simulink model "HornetXII_Challenge"  (R2026a)
settings: Solver=VariableStepAuto  StopTime=300  AbsTol=1e-3  EnableMultiTasking=on
InitFcn:
  | searchHalfSpan = 5;
  | 
  | rng('shuffle');
  | Environment.target.seed = randi(2^31 - 1);
  | 
  | % Use the saved seed to make this particular run reproducible if needed.
  | rng(Environment.target.seed, 'twister');
  | 
  | Environment.target.xy = (2*rand(2,1) - 1) * searchHalfSpan;
  | 
  | Environment.target.pos = [Environment.target.xy;
  |     Environment.seafloordepth - Environment.target.side/2];
values from neighbouring files (symbols this model uses):
  N = size(Vehicle.thrusterori, 2)    [VehicleParameters.m]
undefined symbols (not defined in the file or in its folder): B, pospoints, Spline, timepoints, Vehicle, X, Y, Z
libraries: sm_lib x554, nesl_utility x23, slpidlib x13, matrix_library x4, robotcorelib x2, fl_lib x1, simulink x1
(part 1 of 14)
settings Model: Creator=chesi  LastModifiedBy=kianm
settings DebuggingCC: SubsystemReferenceDiagnosticForUnitTest=warning
settings SimscapeCC: SimscapeNominalValues="[{\"value\":\"1\",\"unit\":\"A\"},{\"value\":\"1\",\"unit\":\"bar\"},{\"value\":\"1\",\"unit\":\"cm^2\"},{\"value\":\"1\",\"unit\":\"cm^3/s\"},{\"value\":\"1\",\"unit\":\"kJ/kg\"},{\"value\":\"1\",\"unit\":\"kW\"},{\"value\":\"1\",\"unit\":\"l\"},{\"value\":\"1\",\"unit\":\"N\"},{\"value\":\"1\",\"unit\":\"N*m\"},{\"value\":\"1\",\"unit\":\"V\"}]"  SimscapeLogSimulationStatistics=on
settings ExplorerConfigSet: InternalSimMechanicsExplorerSettings=|
  | <ExplorerConfiguration>
  | 
  |   <canonicalview>default</canonicalview>
  | 
  |   <TilePanel>
  |     <TileInfo>
  |       <Tiles Columns="2" Count="4" Height="1049" Rows="2" Width="1462">
  |         <Row Weight="0.5"/>
  |         <Row Weight="0.5"/>
  |         <Column Weight="0.5"/>
  |         <Column Weight="0.5"/>
  |         <Tile Height="1" Width="1" X="0" Y="0"/>
  |         <Tile Height="1" Width="1" X="0" Y="1"/>
  |         <Tile Height="1" Width="1" X="1" Y="0"/>
  |         <Tile Height="1" Width="1" X="1" Y="1"/>
  |       </Tiles>
  |     </TileInfo>
  |     <SceneInfo>
  |       <SceneViewer>
  |         <IsThisViewStd>
  |           <IsStandardView>off</IsStandardView>
  |           <StandardViewName>Front</StandardViewName>
  |         </IsThisViewStd>
  |         <BGColor>
  |           <R>1</R>
  |           <G>1</G>
  |           <B>1</B>
  |           <A>1</A>
  |         </BGColor>
  |         <Camera>
  |           <DoPerspective>on</DoPerspective>
  |           <Position>
  |             <X>-1.4139999999999999</X>
  |             <Y>0</Y>
  |             <Z>1</Z>
  |           </Position>
  |           <Center>
  |             <X>0</X>
  |             <Y>0</Y>
  |             <Z>0</Z>
  |           </Center>
  |           <Up>
  |             <X>0.57740839789430587</X>
  |             <Y>0</Y>
  |             <Z>0.81645547462254864</Z>
  |           </Up>
  |           <XLim>0.80758724648884639</XLim>
  |           <YLim>0.80758724648884639</YLim>
  |           <ViewLimDist>0.01</ViewLimDist>
  |         </Camera>
  |       </SceneViewer>
  |       <SceneViewer>
  |         <IsThisViewStd>
  |           <IsStandardView>off</IsStandardView>
  |           <StandardViewName>Front</StandardViewName>
  |         </IsThisViewStd>
  |         <BGColor>
  |           <R>1</R>
  |           <G>1</G>
  |           <B>1</B>
  |           <A>1</A>
  |         </BGColor>
  |         <Camera>
  |           <DoPerspective>on</DoPerspective>
  |           <Position>
  |             <X>0</X>
  |             <Y>0</Y>
  |             <Z>2.5</Z>
  |           </Position>
  |           <Center>
  |             <X>0</X>
  |             <Y>0</Y>
  |             <Z>0</Z>
  |           </Center>
  |           <Up>
  |             <X>1</X>
  |             <Y>0</Y>
  |             <Z>0</Z>
  |           </Up>
  |           <XLim>1.1657691453874972</XLim>
  |           <YLim>1.1657691453874972</YLim>
  |           <ViewLimDist>0.01</ViewLimDist>
  |         </Camera>
  |       </SceneViewer>
  |       <SceneViewer>
  |         <IsThisViewStd>
  |           <IsStandardView>off</IsStandardView>
  |           <StandardViewName>Front</StandardViewName>
  |         </IsThisViewStd>
  |         <BGColor>
  |           <R>1</R>
  |           <G>1</G>
  |           <B>1</B>
  |           <A>1</A>
  |         </BGColor>
  |         <Camera>
  |           <DoPerspective>off</DoPerspective>
  |           <Position>
  |             <X>-0.023481336045726414</X>
  |             <Y>1.0064517868689387</Y>
  |             <Z>83.52507923435725</Z>
  |           </Position>
  |           <Center>
  |             <X>-0.010188562910498078</X>
  |             <Y>1</Y>
  |             <Z>-1.4383130630604528</Z>
  |           </Center>
  |           <Up>
  |             <X>0.99999998774834031</X>
  |             <Y>5.0907915827116125e-06</Y>
  |             <Z>0.00015645255878126614</Z>
  |           </Up>
  |           <XLim>10.310637364602009</XLim>
  |           <YLim>10.310637364602009</YLim>
  |           <ViewLimDist>0.01</ViewLimDist>
  |         </Camera>
  |       </SceneViewer>
  |       <SceneViewer>
  |         <IsThisViewStd>
  |           <IsStandardView>off</IsStandardView>
  |           <StandardViewName>Front</StandardViewName>
  |         </IsThisViewStd>
  |         <BGColor>
  |           <R>1</R>
  |           <G>1</G>
  |           <B>1</B>
  |           <A>1</A>
  |         </BGColor>
  |         <Camera>
  |           <DoPerspective>on</DoPerspective>
  |           <Position>
  |             <X>0</X>
  |             <Y>0</Y>
  |             <Z>-0.25</Z>
  |           </Position>
  |           <Center>
  |             <X>0</X>
  |             <Y>0</Y>
  |             <Z>-1.25</Z>
  |           </Center>
  |           <Up>
  |             <X>1</X>
  |             <Y>0</Y>
  |             <Z>0</Z>
  |           </Up>
  |           <XLim>0.46630765815499897</XLim>
  |           <YLim>0.46630765815499897</YLim>
  |           <ViewLimDist>0.01</ViewLimDist>
  |         </Camera>
  |       </SceneViewer>
  |     </SceneInfo>
  |   </TilePanel>
  | 
  |   <MechEditorPanel>
  |     <GfxPanelCameraMap>
  |       <MapElement CameraMLId="Camera5" GfxPanelIndex="0"/>
  |       <MapElement CameraMLId="Camera7" GfxPanelIndex="1"/>
  |       <MapElement CameraMLId="Camera9" GfxPanelIndex="3"/>
  |     </GfxPanelCameraMap>
  |     <Cameras>
  |       <Camera>
  |         <Id>Camera5</Id>
  |         <Value>
  |           <Name>Behind Up</Name>
  |           <NativeCamera>
  |             <PositionTrackingFeature>Simulator.Cameras.Behind_Up.R</PositionTrackingFeature>
  |             <CenterTrackingFeature>Simulator.AUV_model.BODY</CenterTrackingFeature>
  |             <UpVectorTrackingFeature>Simulator.AUV_model.BODY</UpVectorTrackingFeature>
  |             <CenterTrackingOrigin>on</CenterTrackingOrigin>
  |             <UpVectorTrackingDirection>+X</UpVectorTrackingDirection>
  |           </NativeCamera>
  |         </Value>
  |       </Camera>
  |       <Camera>
  |         <Id>Camera6</Id>
  |         <Value>
  |           <Name>Behind Up Left</Name>
  |           <NativeCamera>
  |             <PositionTrackingFeature>Simulator.Cameras.Behind_Up_Left.R</PositionTrackingFeature>
  |             <CenterTrackingFeature>Simulator.AUV_model.BODY</CenterTrackingFeature>
  |             <UpVectorTrackingFeature>Simulator.AUV_model.BODY</UpVectorTrackingFeature>
  |             <CenterTrackingOrigin>on</CenterTrackingOrigin>
  |             <UpVectorTrackingDirection>-Z</UpVectorTrackingDirection>
  |           </NativeCamera>
  |         </Value>
  |       </Camera>
  |       <Camera>
  |         <Id>Camera7</Id>
  |         <Value>
  |           <Name>Top</Name>
  |           <NativeCamera>
  |             <PositionTrackingFeature>Simulator.Cameras.Top.R</PositionTrackingFeature>
  |             <CenterTrackingFeature>Simulator.AUV_model.BODY</CenterTrackingFeature>
  |             <UpVectorTrackingFeature>Simulator.AUV_model.BODY</UpVectorTrackingFeature>
  |             <CenterTrackingOrigin>on</CenterTrackingOrigin>
  |             <UpVectorTrackingDirection>+X</UpVectorTrackingDirection>
  |           </NativeCamera>
  |         </Value>
  |       </Camera>
  |       <Camera>
  |         <Id>Camera8</Id>
  |         <Value>
  |           <Name>Left</Name>
  |           <NativeCamera>
  |             <PositionTrackingFeature>Simulator.Cameras.Left.R</PositionTrackingFeature>
  |             <CenterTrackingFeature>Simulator.AUV_model.BODY</CenterTrackingFeature>
  |             <UpVectorTrackingFeature>Simulator.AUV_model.BODY</UpVectorTrackingFeature>
  |             <CenterTrackingOrigin>on</CenterTrackingOrigin>
  |             <UpVectorTrackingDirection>-Z</UpVectorTrackingDirection>
  |           </NativeCamera>
  |         </Value>
  |       </Camera>
  |       <Camera>
  |         <Id>Camera9</Id>
  |         <Value>
  |           <Name>BottomCamera</Name>
  |           <NativeCamera>
  |             <PositionTrackingFeature>Simulator.Cameras.Bottom_Camera.R</PositionTrackingFeature>
  |             <CenterTrackingFeature>Simulator.Cameras.Bottom_Camera.R</CenterTrackingFeature>
  |             <UpVectorTrackingFeature>Simulator.Cameras.Bottom_Camera.R</UpVectorTrackingFeature>
  |             <CenterTrackingOrigin>off</CenterTrackingOrigin>
  |             <CenterTrackingDirection>+Z</CenterTrackingDirection>
  |             <UpVectorTrackingDirection>+X</UpVectorTrackingDirection>
  |           </NativeCamera>
  |         </Value>
  |       </Camera>
  |     </Cameras>
  |     <VideoCreator>
  |       <IncludeTiles>All</IncludeTiles>
  |       <IncludeTime>on</IncludeTime>
  |       <IncludeWorldFrame>off</IncludeWorldFrame>
  |       <PlaybackSpeedRatio>1</PlaybackSpeedRatio>
  |       <FrameRate>30</FrameRate>
  |       <FrameSize>auto</FrameSize>
  |       <VideoFormat>UncompressedAVI</VideoFormat>
  |     </VideoCreator>
  |   </MechEditorPanel>
  | 
  |   <PlaybackSettings>
  |     <PlaybackSpeedFactor>2</PlaybackSpeedFactor>
  |   </PlaybackSettings>
  | 
  | </ExplorerConfiguration>

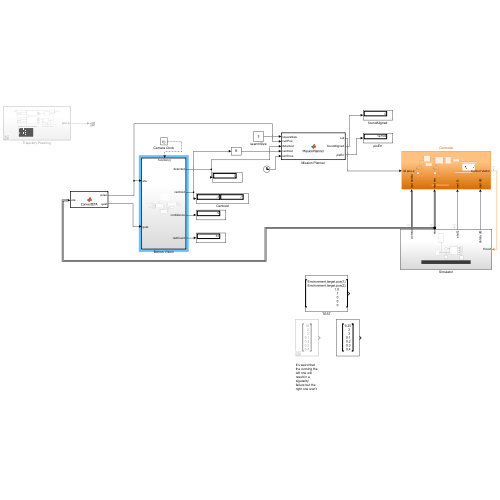
[thumbnail: Simulink's stored preview of the top-level diagram]
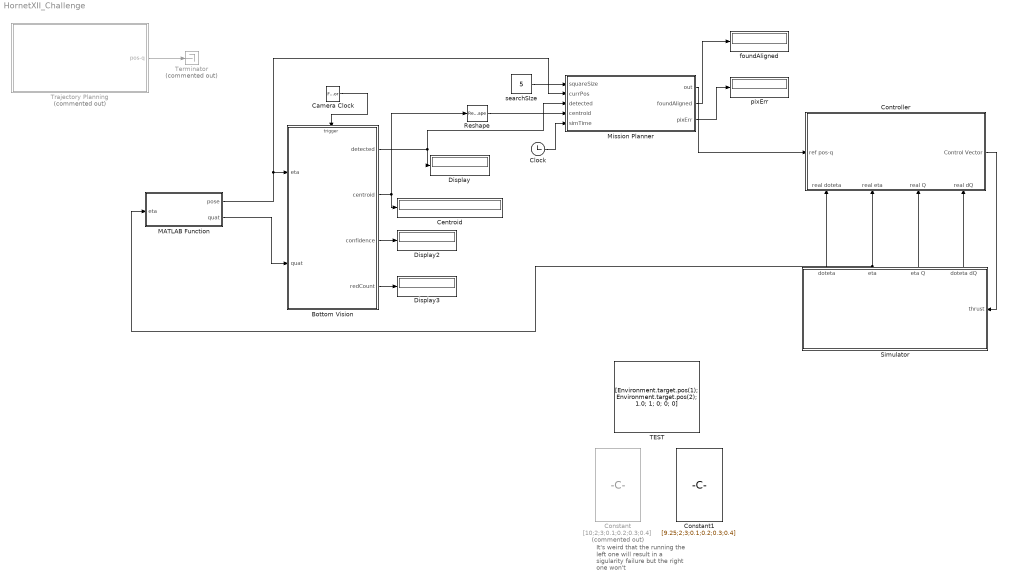
== system HornetXII_Challenge ==
  note: It's weird that the running the left one will result in a sigularity failure but the right one won't
  Bottom Vision : Subsystem  TreatAsAtomicUnit=on
  Camera Clock : FunctionCallGenerator  SampleTime=.2
  Centroid : Display
  Clock : Clock
  Constant : Constant  Commented=on  Value=[10;2;3;0.1;0.2;0.3;0.4]  VectorParams1D=off
  Constant1 : Constant  Value=[9.25;2;3;0.1;0.2;0.3;0.4]  VectorParams1D=off
  Controller : Subsystem
      settings: PortSchema="{\"entries\":[{\"content\":{\"sides\":[{\"content\":{\"connectorIds\":[\"In1\"]},\"type\":\"ConnectorPlacement.EquallySpacedRectSide\",\"uuid\":\"81dc70ea-c00b-487c-98ee-990ff0e578a9\"},{\"content\":{\"connectorIds\":[\"Out1\"],\"side\":\"RIGHT\"},\"type\":\"ConnectorPlacement.EquallySpacedRectSide\",\"uuid\":\"b4d94801-500f-4262-ae87-d28847072c57\"},{\"content\":{\"side\":\"TOP\"},\"type\":\"ConnectorPlacement.EquallySpacedRectSide\",\"uuid\":\"9c8bb19e-0c4f-4865-8be8-8f504c3461c9\"},{\"content\":{\"connectorIds\":[\"In2\",\"In3\",\"In4\",\"In5\"],\"side\":\"BOTTOM\"},\"type\":\"ConnectorPlacement.EquallySpacedRectSide\",\"uuid\":\"42aa0f8d-cdff-4cb2-b13b-82c7b92e497b\"}]},\"type\":\"ConnectorPlacement.EquallySpacedConnector\",\"uuid\":\"3d0765d3-7e16-47e0-887a-613e0e5dbe32\"}],\"packageUris\":[\"http://schema.mathworks.com/mf0/Connector/R2020b\"],\"version\":\"1.0\"}"
  Display : Display
  Display2 : Display
  Display3 : Display
  MATLAB Function : MATLAB Function  TreatAsAtomicUnit=on
  Mission Planner : MATLAB Function  TreatAsAtomicUnit=on
  Reshape : Reshape  OutputDimensionality=Customize  OutputDimensions=[2,1]
  Simulator : Subsystem
      settings: PortSchema="{\"entries\":[{\"content\":{\"sides\":[{\"content\":{\"connectorIds\":[\"In1\"]},\"type\":\"ConnectorPlacement.EquallySpacedRectSide\",\"uuid\":\"7f0b7788-e8a3-4936-9374-02ac1b67f663\"},{\"content\":{\"side\":\"RIGHT\"},\"type\":\"ConnectorPlacement.EquallySpacedRectSide\",\"uuid\":\"45623c25-ae9c-4192-a7b0-dfa9bedf06ea\"},{\"content\":{\"connectorIds\":[\"Out1\",\"Out2\",\"Out3\",\"Out4\"],\"side\":\"TOP\"},\"type\":\"ConnectorPlacement.EquallySpacedRectSide\",\"uuid\":\"6471b253-20e0-4344-8e89-5b5e84cfa395\"},{\"content\":{\"side\":\"BOTTOM\"},\"type\":\"ConnectorPlacement.EquallySpacedRectSide\",\"uuid\":\"e37f05fa-5476-47a4-acd2-111dd632b18c\"}]},\"type\":\"ConnectorPlacement.EquallySpacedConnector\",\"uuid\":\"72a4f9be-cf7b-4481-94c8-675ac13ca12c\"}],\"packageUris\":[\"http://schema.mathworks.com/mf0/Connector/R2020b\"],\"version\":\"1.0\"}"
  TEST : Constant  Value=|  VectorParams1D=off
      | [Environment.target.pos(1);
      |  Environment.target.pos(2);
      |  1.0;
      |  1;
      |  0;
      |  0;
      |  0]
  Terminator : Terminator  Commented=on
  Trajectory Planning : Subsystem  Commented=on
  foundAligned : Display
  pixErr : Display
  searchSIze : Constant  Value=5
  wires:
  searchSIze/1 -> Mission Planner/1(squareSize)
  Trajectory Planning/1(pos-q) -> Terminator/1
  Simulator/4(doteta) -> Controller/2(real doteta)
  Simulator/2(eta Q) -> Controller/4(real Q)
  MATLAB Function/2(quat) -> Bottom Vision/2(quat)
  Simulator/3(eta) -> Controller/3(real eta), MATLAB Function/1(eta)
  Simulator/1(doteta dQ) -> Controller/5(real dQ)
  Camera Clock/1 -> Bottom Vision/Trigger
  MATLAB Function/1(pose) -> Mission Planner/2(currPos), Bottom Vision/1(eta)
  Bottom Vision/3(confidence) -> Display2/1
  Bottom Vision/1(detected) -> Mission Planner/3(detected), Display/1
  Bottom Vision/4(redCount) -> Display3/1
  Bottom Vision/2(centroid) -> Reshape/1, Centroid/1
  Reshape/1 -> Mission Planner/4(centroid)
  Clock/1 -> Mission Planner/5(simTime)
  Mission Planner/1(out) -> Controller/1(ref pos-q)
  Mission Planner/2(foundAligned) -> foundAligned/1
  Mission Planner/3(pixErr) -> pixErr/1
  Controller/1(Control Vector) -> Simulator/1(thrust)

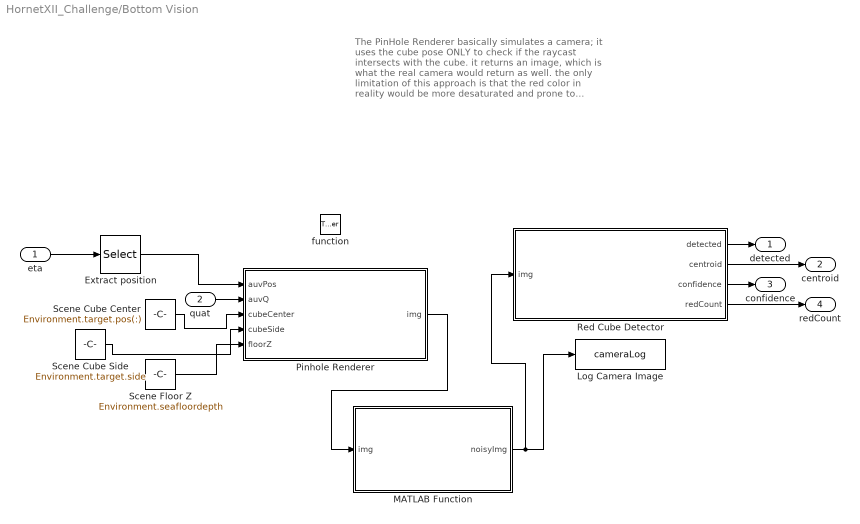
== system HornetXII_Challenge/Bottom Vision ==
  note: The PinHole Renderer basically simulates a camera; it uses the cube pose ONLY to check if the raycast intersects with the cube. it returns an image, which is what the real camera would return as well. the only limitation of this approach is that the red color in reality would be more desaturated and prone to interferences. I have added a simple noise layer, but I think this part of the simulation could be made more realistic by processing the image to be more like the underwater conditions
  eta : Inport
  quat : Inport  Port=2
  function : TriggerPort  TriggerType=function-call  VariantControl=(inherit)
  Extract position : Selector  InputPortWidth=3  IndexOptions=Index vector (dialog)  Indices=[1 2 3]  OutputSizes=1
  Log Camera Image : ToWorkspace  VariableName=cameraLog  SaveFormat=Structure With Time  SampleTime=-1
      settings: MaxDataPoints=500
  MATLAB Function : MATLAB Function  TreatAsAtomicUnit=on
  Pinhole Renderer : MATLAB Function  TreatAsAtomicUnit=on
  Red Cube Detector : MATLAB Function  TreatAsAtomicUnit=on
  Scene Cube Center : Constant  Value=Environment.target.pos(:)
  Scene Cube Side : Constant  Value=Environment.target.side
  Scene Floor Z : Constant  Value=Environment.seafloordepth
  detected : Outport
  centroid : Outport  Port=2
  confidence : Outport  Port=3
  redCount : Outport  Port=4
  wires:
  eta/1 -> Extract position/1
  Extract position/1 -> Pinhole Renderer/1(auvPos)
  quat/1 -> Pinhole Renderer/2(auvQ)
  Scene Cube Center/1 -> Pinhole Renderer/3(cubeCenter)
  Scene Cube Side/1 -> Pinhole Renderer/4(cubeSide)
  Scene Floor Z/1 -> Pinhole Renderer/5(floorZ)
  Pinhole Renderer/1(img) -> MATLAB Function/1(img)
  Red Cube Detector/1(detected) -> detected/1
  Red Cube Detector/2(centroid) -> centroid/1
  Red Cube Detector/3(confidence) -> confidence/1
  Red Cube Detector/4(redCount) -> redCount/1
  MATLAB Function/1(noisyImg) -> Red Cube Detector/1(img), Log Camera Image/1

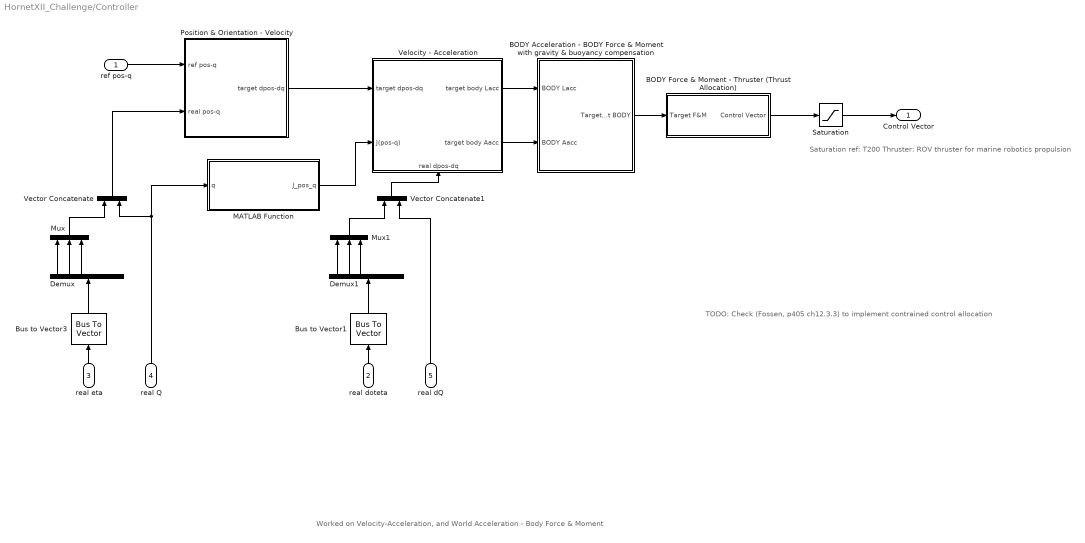
== system HornetXII_Challenge/Controller ==
  note: Saturation ref: T200 Thruster: ROV thruster for marine robotics propulsion
  note: Worked on Velocity-Acceleration, and World Acceleration - Body Force & Moment
  note: TODO: Check (Fossen, p405 ch12.3.3) to implement contrained control allocation
  ref pos-q : Inport
  real doteta : Inport  Port=2
  real eta : Inport  Port=3
  real Q : Inport  Port=4
  real dQ : Inport  Port=5
  BODY Acceleration - BODY Force & Moment with gravity & buoyancy compensation : Subsystem
  BODY Force & Moment - Thruster (Thrust Allocation) : Subsystem
  Bus to Vector1 : BusToVector
  Bus to Vector3 : BusToVector
  Demux : Demux  Outputs=6
  Demux1 : Demux  Outputs=6
  MATLAB Function : MATLAB Function  TreatAsAtomicUnit=on
  Mux : Mux  Inputs=3
  Mux1 : Mux  Inputs=3
  Position & Orientation - Velocity : Subsystem
  Saturation : Saturate  UpperLimit=50  LowerLimit=-40
  Vector Concatenate : Concatenate
  Vector Concatenate1 : Concatenate
  Velocity - Acceleration : Subsystem
      settings: PortSchema="{\"entries\":[{\"content\":{\"sides\":[{\"content\":{\"connectorIds\":[\"In1\",\"In2\"]},\"type\":\"ConnectorPlacement.EquallySpacedRectSide\",\"uuid\":\"ee3a7c6d-14b0-4eab-a7d5-084df5aecf6b\"},{\"content\":{\"connectorIds\":[\"Out1\",\"Out2\"],\"side\":\"RIGHT\"},\"type\":\"ConnectorPlacement.EquallySpacedRectSide\",\"uuid\":\"abac75c8-6f4b-4c3d-963c-0e4665da2ede\"},{\"content\":{\"side\":\"TOP\"},\"type\":\"ConnectorPlacement.EquallySpacedRectSide\",\"uuid\":\"57e3df7e-6308-4dbd-864e-1b3862b04628\"},{\"content\":{\"connectorIds\":[\"In3\"],\"side\":\"BOTTOM\"},\"type\":\"ConnectorPlacement.EquallySpacedRectSide\",\"uuid\":\"98abef76-2ed0-406f-af2c-887e86df641b\"}]},\"type\":\"ConnectorPlacement.EquallySpacedConnector\",\"uuid\":\"1e3d0704-0b7c-47be-86c5-b073cfbb5b69\"}],\"packageUris\":[\"http://schema.mathworks.com/mf0/Connector/R2020b\"],\"version\":\"1.0\"}"
  Control Vector : Outport
  wires:
  ref pos-q/1 -> Position & Orientation - Velocity/1(ref pos-q)
  BODY Acceleration - BODY Force & Moment with gravity & buoyancy compensation/1(Target F&M at BODY) -> BODY Force & Moment - Thruster (Thrust Allocation)/1(Target F&M)
  Velocity - Acceleration/2(target body Aacc) -> BODY Acceleration - BODY Force & Moment with gravity & buoyancy compensation/2(BODY Aacc)
  Velocity - Acceleration/1(target body Lacc) -> BODY Acceleration - BODY Force & Moment with gravity & buoyancy compensation/1(BODY Lacc)
  real eta/1 -> Bus to Vector3/1
  BODY Force & Moment - Thruster (Thrust Allocation)/1(Control Vector) -> Saturation/1
  Saturation/1 -> Control Vector/1
  Bus to Vector3/1 -> Demux/1
  Mux/1 -> Vector Concatenate/1
  real Q/1 -> Vector Concatenate/2, MATLAB Function/1(q)
  Vector Concatenate/1 -> Position & Orientation - Velocity/2(real pos-q)
  Bus to Vector1/1 -> Demux1/1
  real doteta/1 -> Bus to Vector1/1
  real dQ/1 -> Vector Concatenate1/2
  Position & Orientation - Velocity/1(target dpos-dq) -> Velocity - Acceleration/1(target dpos-dq)
  MATLAB Function/1(J_pos_q) -> Velocity - Acceleration/2(J(pos-q))
  Vector Concatenate1/1 -> Velocity - Acceleration/3(real dpos-dq)
  Demux/1 -> Mux/1
  Demux/2 -> Mux/2
  Demux/3 -> Mux/3
  Demux1/1 -> Mux1/1
  Demux1/2 -> Mux1/2
  Demux1/3 -> Mux1/3
  Mux1/1 -> Vector Concatenate1/1

== system HornetXII_Challenge/Simulator ==
  thrust : Inport
  AUV model : Subsystem
  Cameras : Subsystem
  NED-Seafloor : sm_lib/Frames and Transforms/Rigid Transform  RotationMethod=None  FollAlignAxisA=-Z  BaseAlignAxisA=+Z  FollAlignAxisB=+X  BaseAlignAxisB=+X  RotationStandardAxis=+Z  RotationAngle=0.0  RotationAngleUnits=deg  RotationArbitraryAxis=[0 0 1]  RotationSequenceAxes=FollowerAxes  RotationSequence=XYX  RotationSequenceAngles=[0 0 0]  RotationSequenceAnglesUnits=deg  RotationMatrix=[1 0 0; 0 1 0; 0 0 1]  Quaternion=[1 0 0 0]  TranslationMethod=Cartesian  TranslationCartesianOffset=[-Environment.seafloortileside*5 0 Environment.seafloordepth]  TranslationCartesianOffsetUnits=m  TranslationStandardAxis=+Z  TranslationStandardOffset=0  TranslationStandardOffsetUnits=m  TranslationROffset=0  TranslationROffsetUnits=m  TranslationThetaOffset=0  TranslationThetaOffsetUnits=deg  TranslationZOffset=0  TranslationZOffsetUnits=m
  Target Object : Subsystem
  Tiled Seafloor : Subsystem  mask(Tiled Grid){side=Environment.seafloortileside, thick=0.004, color1=[0 0.8 0.4], color2=[0 0.6 0.8], opacity=1}
      mask prompts: side "Tile Side (m) :"; thick "Tile Thickness (m) :"; color1 "First Color [RGB] :"; color2 "Second Color [RGB] :"; opacity "Tile Opacity (0...1) :"
      mask help: This block creates a tiled grid composed of square tiles.
  World : Subsystem
  doteta dQ : Outport
  eta Q : Outport  Port=2
  eta : Outport  Port=3
  doteta : Outport  Port=4
  wires:
  thrust/1 -> AUV model/1(thrust)
  AUV model/2(eta) -> eta/1
  AUV model/1(doteta) -> doteta/1
  AUV model/3(eta Q) -> eta Q/1
  AUV model/4(doteta dQ) -> doteta dQ/1
  connections:
  Tiled Seafloor/LConn1 -- NED-Seafloor/RConn1
  AUV model/RConn1 -- Cameras/LConn1
  AUV model/LConn1 -- World/RConn1 -- Target Object/LConn1 -- NED-Seafloor/LConn1

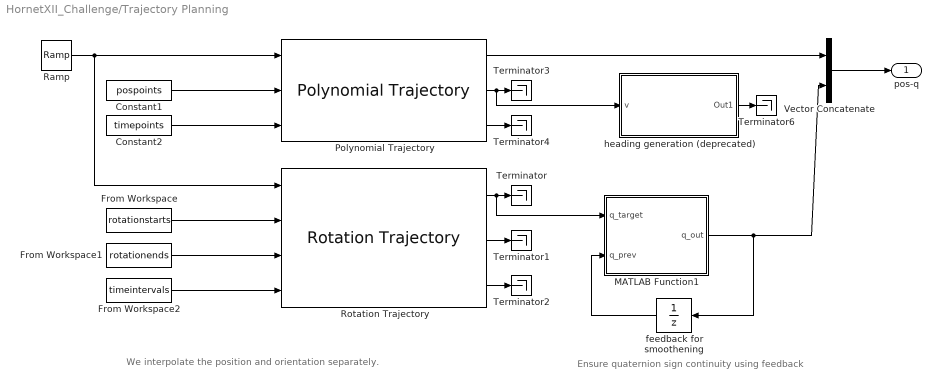
== system HornetXII_Challenge/Trajectory Planning ==
  note: Ensure quaternion sign continuity using feedback
  note: We interpolate the position and orientation separately.
  Constant1 : Constant  Value=pospoints
  Constant2 : Constant  Value=timepoints
  From Workspace : FromWorkspace  VariableName=rotationstarts  Interpolate=off  OutputAfterFinalValue=Holding final value
  From Workspace1 : FromWorkspace  VariableName=rotationends  Interpolate=off  OutputAfterFinalValue=Holding final value
  From Workspace2 : FromWorkspace  VariableName=timeintervals  Interpolate=off  OutputAfterFinalValue=Holding final value
  MATLAB Function1 : MATLAB Function  TreatAsAtomicUnit=on
  Polynomial Trajectory : robotcorelib/Polynomial Trajectory  WaypointSource=External  Waypoints=pospoints  TimePoints=timepoints  TimeInterval=[ 1, 4 ]  Method=B-Spline  ParameterSource=Internal  VelocityBoundaryCondition=zeros(3,5)  AccelerationBoundaryCondition=zeros( 2, 5 )  SimulateUsing=Interpreted execution
  Ramp : simulink/Sources/Ramp  slope=1  start=0  InitialOutput=0
  Rotation Trajectory : robotcorelib/Rotation Trajectory  WaypointFormat=Quaternion  WaypointSource=External  R0=[ 1, 0, 0, 0 ]'  RF=[ 0, 0, 1, 0 ]'  TimeInterval=[ 0, 1 ]  CustomTimeScaling=off  ParameterSource=Internal  TSTime=0:0.1:1  TimeScaling=[ 0:0.1:1; ones( 1, 11 ); zeros( 1, 11 ) ]  SimulateUsing=Interpreted execution
      settings: LibrarySourceBlock=robotutilslib/Rotation Trajectory
  Terminator{,1..4,6} (6 alike) : Terminator
  Vector Concatenate : Concatenate
  feedback for smoothening : UnitDelay  InitialCondition=[1 0 0 0]'  SampleTime=0.5
  heading generation (deprecated) : Subsystem
  pos-q : Outport
  wires:
  From Workspace2/1 -> Rotation Trajectory/4
  MATLAB Function1/1(q_out) -> feedback for smoothening/1, Vector Concatenate/2
  Rotation Trajectory/2 -> Terminator1/1
  Polynomial Trajectory/1 -> Vector Concatenate/1
  Constant1/1 -> Polynomial Trajectory/2
  Ramp/1 -> Polynomial Trajectory/1, Rotation Trajectory/1
  From Workspace/1 -> Rotation Trajectory/2
  From Workspace1/1 -> Rotation Trajectory/3
  feedback for smoothening/1 -> MATLAB Function1/2(q_prev)
  Rotation Trajectory/1 -> MATLAB Function1/1(q_target), Terminator/1
  Polynomial Trajectory/2 -> heading generation (deprecated)/1(v), Terminator3/1
  Constant2/1 -> Polynomial Trajectory/3
  heading generation (deprecated)/1(Out1) -> Terminator6/1
  Rotation Trajectory/3 -> Terminator2/1
  Polynomial Trajectory/3 -> Terminator4/1
  Vector Concatenate/1 -> pos-q/1

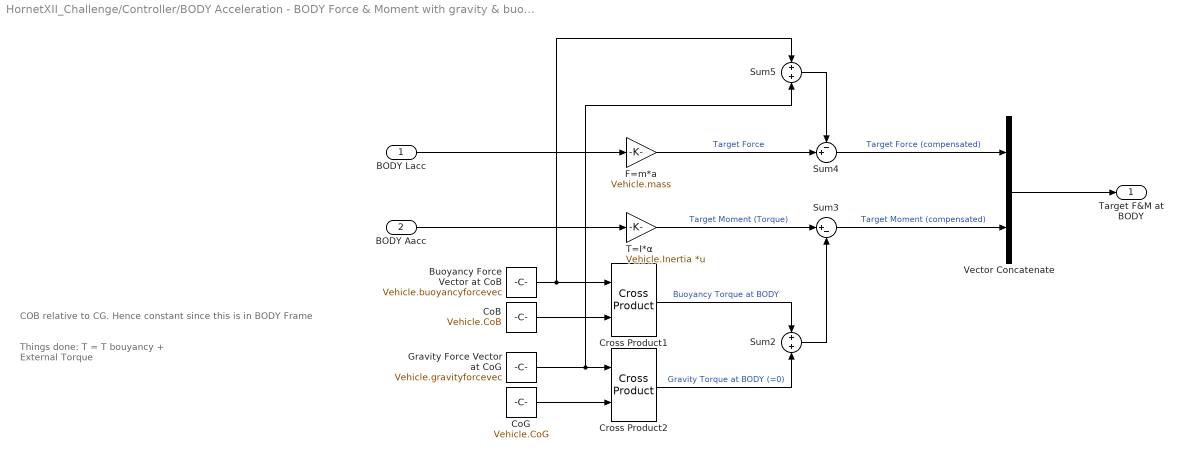
== system HornetXII_Challenge/Controller/BODY Acceleration - BODY Force & Moment with gravity & buoyancy compensation ==
  note: COB relative to CG. Hence constant since this is in BODY Frame
  note: Things done:
      | T = T bouyancy + External Torque
  BODY Lacc : Inport
  BODY Aacc : Inport  Port=2
  Buoyancy Force Vector at CoB : Constant  Value=Vehicle.buoyancyforcevec
  CoB : Constant  Value=Vehicle.CoB
  CoG : Constant  Value=Vehicle.CoG
  Cross Product1 : matrix_library/Cross Product
  Cross Product2 : matrix_library/Cross Product
  F=m*a : Gain  Gain=Vehicle.mass
  Gravity Force Vector at CoG : Constant  Value=Vehicle.gravityforcevec
  Sum2 : Sum  Inputs=+|+
  Sum3 : Sum  Inputs=|+-
  Sum4 : Sum  Inputs=-+|
  Sum5 : Sum  Inputs=+|+
  T=I*α : Gain  Gain=Vehicle.Inertia  Multiplication=Matrix(K*u)
  Vector Concatenate : Concatenate
  Target F&M at BODY : Outport
  wires:
  Vector Concatenate/1 -> Target F&M at BODY/1
  CoB/1 -> Cross Product1/2
  BODY Lacc/1 -> F=m*a/1
  BODY Aacc/1 -> T=I*α/1
  T=I*α/1 -> Sum3/1  "Target Moment (Torque)"
  Sum3/1 -> Vector Concatenate/2  "Target Moment (compensated)"
  F=m*a/1 -> Sum4/2  "Target Force"
  Sum4/1 -> Vector Concatenate/1  "Target Force (compensated)"
  Buoyancy Force Vector at CoB/1 -> Cross Product1/1, Sum5/1
  Gravity Force Vector at CoG/1 -> Cross Product2/1, Sum5/2
  CoG/1 -> Cross Product2/2
  Cross Product1/1 -> Sum2/1  "Buoyancy Torque at BODY"
  Cross Product2/1 -> Sum2/2  "Gravity Torque at BODY (=0)"
  Sum2/1 -> Sum3/2
  Sum5/1 -> Sum4/1

== system HornetXII_Challenge/Controller/BODY Force & Moment - Thruster (Thrust Allocation) ==
  Target F&M : Inport
  Thrust Alloc. Matrix : Gain  Gain=Vehicle.thrustallocmatrix  Multiplication=Matrix(K*u)
  Control Vector : Outport
  wires:
  Target F&M/1 -> Thrust Alloc. Matrix/1
  Thrust Alloc. Matrix/1 -> Control Vector/1

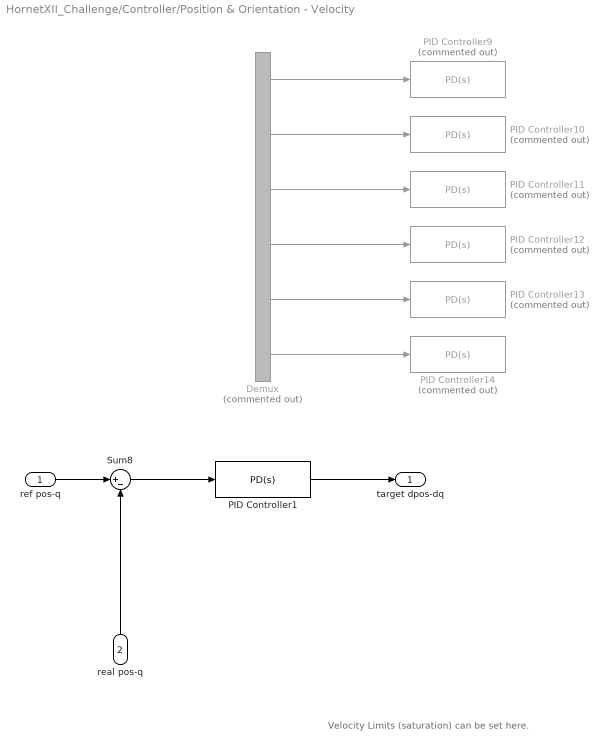
== system HornetXII_Challenge/Controller/Position & Orientation - Velocity ==
  note: Velocity Limits (saturation) can be set here.
  ref pos-q : Inport
  real pos-q : Inport  Port=2
  Demux : Demux  Commented=on  Outputs=6
  PID Controller1 : slpidlib/PID Controller  Controller=PD  Form=Parallel  TimeDomain=Continuous-time  UseExternalTs=off  SampleTime=0.1  IntegratorMethod=Forward Euler  FilterMethod=Forward Euler  ControllerParametersSource=internal  P=1  I=1  UseKiTs=off  D=1  UseExternalDerivativeSource=off  N=200  UseFilter=on  TunerSelectOption=Transfer Function Based (PID Tuner App)  InitialConditionSource=internal  InitialConditionForIntegrator=0  InitialConditionForFilter=0  DifferentiatorICPrevScaledInput=0  ExternalReset=none  TrackingMode=off  Kt=1  LimitOutput=on  SatLimitsSource=internal  UpperSaturationLimit=5  LowerSaturationLimit=-5  LinearizeAsGain=on  AntiWindupMode=none  Kb=1  LimitIntegrator=off  UpperIntegratorSaturationLimit=inf  LowerIntegratorSaturationLimit=-inf  POutMin=[]  POutMax=[]  IOutMin=[]  IOutMax=[]  DOutMin=[]  DOutMax=[]  NOutMin=[]  NOutMax=[]  SumOutMin=[]  SumOutMax=[]  SaturationOutMin=[]  SaturationOutMax=[]  PParamMin=[]  PParamMax=[]  IParamMin=[]  IParamMax=[]  DParamMin=[]  DParamMax=[]  NParamMin=[]  NParamMax=[]  KbParamMin=[]  KbParamMax=[]  KtParamMin=[]  KtParamMax=[]  KbOutMin=[]  KbOutMax=[]  KtOutMin=[]  KtOutMax=[]  IntegratorOutMin=[]  IntegratorOutMax=[]  FilterOutMin=[]  FilterOutMax=[]  SumI1OutMin=[]  SumI1OutMax=[]  SumI2OutMin=[]  SumI2OutMax=[]  SumI3OutMin=[]  SumI3OutMax=[]  SumI4OutMin=[]  SumI4OutMax=[]  SumDOutMin=[]  SumDOutMax=[]  DifferentiatorOutMin=[]  DifferentiatorOutMax=[]  FilterDiffOutCoefMin=[]  FilterDiffOutCoefMax=[]  ReciprocalOutMin=[]  ReciprocalOutMax=[]  SumDenOutMin=[]  SumDenOutMax=[]  SumNumOutMin=[]  SumNumOutMax=[]  DivideOutMin=[]  DivideOutMax=[]  UdiffTsProdOutMin=[]  UdiffTsProdOutMax=[]  NTsProdOutMin=[]  NTsProdOutMax=[]  UintegralTsProdOutMin=[]  UintegralTsProdOutMax=[]  UngainTsProdOutMin=[]  UngainTsProdOutMax=[]  ClampingZeroOutDataTypeStr=Inherit: Inherit via back propagation  ClampingZeroOutMin=[]  ClampingZeroOutMax=[]  FilterDenConstantOutDataTypeStr=Inherit: Inherit via back propagation  FilterDenConstantOutMin=[]  FilterDenConstantOutMax=[]  PCopyOutDataTypeStr=Inherit: Inherit via back propagation  PCopyOutMin=[]  PCopyOutMax=[]  NCopyOutDataTypeStr=Inherit: Inherit via back propagation  NCopyOutMin=[]  NCopyOutMax=[]  IntegratorContinuousStateAttributes=''  IntegratorStateMustResolveToSignalObject=off  IntegratorRTWStateStorageClass=Auto  FilterContinuousStateAttributes=''  FilterStateMustResolveToSignalObject=off  FilterRTWStateStorageClass=Auto  ParallelPVariant=InternalParameters  IdealPVariant=Disabled  IVariant=Disabled  DVariant=InternalParameters  IntegratorVariant=Disabled  SatVariant=Enabled  AWVariant=Disabled  PCopyVariant=Disabled  TRVariant=Disabled  FdbkBlocksVariant=Forward  IdealPFdbkVariant=Disabled  SatFdbkVariant=Disabled  DerivativeFilterVariant=ContFilter  NVariant=InternalParameters  NCopyVariant=Disabled  FilterICVariant=InternalICsFilter  IntegratorICVariant=Disabled  ExternalResetVariant=Disabled  TRSumVariant=Passthrough  SumFdbkVariant=Disabled  SumVariant=Sum_PD  TsampFilterVariant=InternalTs  TsampNgainVariant=Passthrough  TsampIntegralVariant=Disabled_SignalSpec  ExternalSaturationOutDataTypeStr=Inherit: Same as second input  DerivativeSourceVariant=ErrorSignal  PreIntVariant=InternalPreInt
  PID Controller10 : slpidlib/PID Controller  Commented=on  Controller=PD  Form=Parallel  TimeDomain=Continuous-time  UseExternalTs=off  SampleTime=-1  IntegratorMethod=Forward Euler  FilterMethod=Forward Euler  ControllerParametersSource=internal  P=1  I=1  UseKiTs=off  D=1  UseExternalDerivativeSource=off  N=200  UseFilter=on  TunerSelectOption=Transfer Function Based (PID Tuner App)  InitialConditionSource=internal  InitialConditionForIntegrator=0  InitialConditionForFilter=0  DifferentiatorICPrevScaledInput=0  ExternalReset=none  TrackingMode=off  Kt=1  LimitOutput=on  SatLimitsSource=internal  UpperSaturationLimit=1  LowerSaturationLimit=-1  LinearizeAsGain=on  AntiWindupMode=none  Kb=1  LimitIntegrator=off  UpperIntegratorSaturationLimit=inf  LowerIntegratorSaturationLimit=-inf  POutMin=[]  POutMax=[]  IOutMin=[]  IOutMax=[]  DOutMin=[]  DOutMax=[]  NOutMin=[]  NOutMax=[]  SumOutMin=[]  SumOutMax=[]  SaturationOutMin=[]  SaturationOutMax=[]  PParamMin=[]  PParamMax=[]  IParamMin=[]  IParamMax=[]  DParamMin=[]  DParamMax=[]  NParamMin=[]  NParamMax=[]  KbParamMin=[]  KbParamMax=[]  KtParamMin=[]  KtParamMax=[]  KbOutMin=[]  KbOutMax=[]  KtOutMin=[]  KtOutMax=[]  IntegratorOutMin=[]  IntegratorOutMax=[]  FilterOutMin=[]  FilterOutMax=[]  SumI1OutMin=[]  SumI1OutMax=[]  SumI2OutMin=[]  SumI2OutMax=[]  SumI3OutMin=[]  SumI3OutMax=[]  SumI4OutMin=[]  SumI4OutMax=[]  SumDOutMin=[]  SumDOutMax=[]  DifferentiatorOutMin=[]  DifferentiatorOutMax=[]  FilterDiffOutCoefMin=[]  FilterDiffOutCoefMax=[]  ReciprocalOutMin=[]  ReciprocalOutMax=[]  SumDenOutMin=[]  SumDenOutMax=[]  SumNumOutMin=[]  SumNumOutMax=[]  DivideOutMin=[]  DivideOutMax=[]  UdiffTsProdOutMin=[]  UdiffTsProdOutMax=[]  NTsProdOutMin=[]  NTsProdOutMax=[]  UintegralTsProdOutMin=[]  UintegralTsProdOutMax=[]  UngainTsProdOutMin=[]  UngainTsProdOutMax=[]  ClampingZeroOutDataTypeStr=Inherit: Inherit via back propagation  ClampingZeroOutMin=[]  ClampingZeroOutMax=[]  FilterDenConstantOutDataTypeStr=Inherit: Inherit via back propagation  FilterDenConstantOutMin=[]  FilterDenConstantOutMax=[]  PCopyOutDataTypeStr=Inherit: Inherit via back propagation  PCopyOutMin=[]  PCopyOutMax=[]  NCopyOutDataTypeStr=Inherit: Inherit via back propagation  NCopyOutMin=[]  NCopyOutMax=[]  IntegratorContinuousStateAttributes=''  IntegratorStateMustResolveToSignalObject=off  IntegratorRTWStateStorageClass=Auto  FilterContinuousStateAttributes=''  FilterStateMustResolveToSignalObject=off  FilterRTWStateStorageClass=Auto  ParallelPVariant=InternalParameters  IdealPVariant=Disabled  IVariant=Disabled  DVariant=InternalParameters  IntegratorVariant=Disabled  SatVariant=Enabled  AWVariant=Disabled  PCopyVariant=Disabled  TRVariant=Disabled  FdbkBlocksVariant=Forward  IdealPFdbkVariant=Disabled  SatFdbkVariant=Disabled  DerivativeFilterVariant=ContFilter  NVariant=InternalParameters  NCopyVariant=Disabled  FilterICVariant=InternalICsFilter  IntegratorICVariant=Disabled  ExternalResetVariant=Disabled  TRSumVariant=Passthrough  SumFdbkVariant=Disabled  SumVariant=Sum_PD  TsampFilterVariant=InternalTs  TsampNgainVariant=Passthrough  TsampIntegralVariant=Disabled_SignalSpec  ExternalSaturationOutDataTypeStr=Inherit: Same as second input  DerivativeSourceVariant=ErrorSignal  PreIntVariant=InternalPreInt
  PID Controller11 : slpidlib/PID Controller  Commented=on  Controller=PD  Form=Parallel  TimeDomain=Continuous-time  UseExternalTs=off  SampleTime=-1  IntegratorMethod=Forward Euler  FilterMethod=Forward Euler  ControllerParametersSource=internal  P=1  I=1  UseKiTs=off  D=1  UseExternalDerivativeSource=off  N=200  UseFilter=on  TunerSelectOption=Transfer Function Based (PID Tuner App)  InitialConditionSource=internal  InitialConditionForIntegrator=0  InitialConditionForFilter=0  DifferentiatorICPrevScaledInput=0  ExternalReset=none  TrackingMode=off  Kt=1  LimitOutput=on  SatLimitsSource=internal  UpperSaturationLimit=1  LowerSaturationLimit=-1  LinearizeAsGain=on  AntiWindupMode=none  Kb=1  LimitIntegrator=off  UpperIntegratorSaturationLimit=inf  LowerIntegratorSaturationLimit=-inf  POutMin=[]  POutMax=[]  IOutMin=[]  IOutMax=[]  DOutMin=[]  DOutMax=[]  NOutMin=[]  NOutMax=[]  SumOutMin=[]  SumOutMax=[]  SaturationOutMin=[]  SaturationOutMax=[]  PParamMin=[]  PParamMax=[]  IParamMin=[]  IParamMax=[]  DParamMin=[]  DParamMax=[]  NParamMin=[]  NParamMax=[]  KbParamMin=[]  KbParamMax=[]  KtParamMin=[]  KtParamMax=[]  KbOutMin=[]  KbOutMax=[]  KtOutMin=[]  KtOutMax=[]  IntegratorOutMin=[]  IntegratorOutMax=[]  FilterOutMin=[]  FilterOutMax=[]  SumI1OutMin=[]  SumI1OutMax=[]  SumI2OutMin=[]  SumI2OutMax=[]  SumI3OutMin=[]  SumI3OutMax=[]  SumI4OutMin=[]  SumI4OutMax=[]  SumDOutMin=[]  SumDOutMax=[]  DifferentiatorOutMin=[]  DifferentiatorOutMax=[]  FilterDiffOutCoefMin=[]  FilterDiffOutCoefMax=[]  ReciprocalOutMin=[]  ReciprocalOutMax=[]  SumDenOutMin=[]  SumDenOutMax=[]  SumNumOutMin=[]  SumNumOutMax=[]  DivideOutMin=[]  DivideOutMax=[]  UdiffTsProdOutMin=[]  UdiffTsProdOutMax=[]  NTsProdOutMin=[]  NTsProdOutMax=[]  UintegralTsProdOutMin=[]  UintegralTsProdOutMax=[]  UngainTsProdOutMin=[]  UngainTsProdOutMax=[]  ClampingZeroOutDataTypeStr=Inherit: Inherit via back propagation  ClampingZeroOutMin=[]  ClampingZeroOutMax=[]  FilterDenConstantOutDataTypeStr=Inherit: Inherit via back propagation  FilterDenConstantOutMin=[]  FilterDenConstantOutMax=[]  PCopyOutDataTypeStr=Inherit: Inherit via back propagation  PCopyOutMin=[]  PCopyOutMax=[]  NCopyOutDataTypeStr=Inherit: Inherit via back propagation  NCopyOutMin=[]  NCopyOutMax=[]  IntegratorContinuousStateAttributes=''  IntegratorStateMustResolveToSignalObject=off  IntegratorRTWStateStorageClass=Auto  FilterContinuousStateAttributes=''  FilterStateMustResolveToSignalObject=off  FilterRTWStateStorageClass=Auto  ParallelPVariant=InternalParameters  IdealPVariant=Disabled  IVariant=Disabled  DVariant=InternalParameters  IntegratorVariant=Disabled  SatVariant=Enabled  AWVariant=Disabled  PCopyVariant=Disabled  TRVariant=Disabled  FdbkBlocksVariant=Forward  IdealPFdbkVariant=Disabled  SatFdbkVariant=Disabled  DerivativeFilterVariant=ContFilter  NVariant=InternalParameters  NCopyVariant=Disabled  FilterICVariant=InternalICsFilter  IntegratorICVariant=Disabled  ExternalResetVariant=Disabled  TRSumVariant=Passthrough  SumFdbkVariant=Disabled  SumVariant=Sum_PD  TsampFilterVariant=InternalTs  TsampNgainVariant=Passthrough  TsampIntegralVariant=Disabled_SignalSpec  ExternalSaturationOutDataTypeStr=Inherit: Same as second input  DerivativeSourceVariant=ErrorSignal  PreIntVariant=InternalPreInt
  PID Controller12 : slpidlib/PID Controller  Commented=on  Controller=PD  Form=Parallel  TimeDomain=Continuous-time  UseExternalTs=off  SampleTime=-1  IntegratorMethod=Forward Euler  FilterMethod=Forward Euler  ControllerParametersSource=internal  P=1  I=1  UseKiTs=off  D=1  UseExternalDerivativeSource=off  N=200  UseFilter=on  TunerSelectOption=Transfer Function Based (PID Tuner App)  InitialConditionSource=internal  InitialConditionForIntegrator=0  InitialConditionForFilter=0  DifferentiatorICPrevScaledInput=0  ExternalReset=none  TrackingMode=off  Kt=1  LimitOutput=on  SatLimitsSource=internal  UpperSaturationLimit=0.5  LowerSaturationLimit=-0.5  LinearizeAsGain=on  AntiWindupMode=none  Kb=1  LimitIntegrator=off  UpperIntegratorSaturationLimit=inf  LowerIntegratorSaturationLimit=-inf  POutMin=[]  POutMax=[]  IOutMin=[]  IOutMax=[]  DOutMin=[]  DOutMax=[]  NOutMin=[]  NOutMax=[]  SumOutMin=[]  SumOutMax=[]  SaturationOutMin=[]  SaturationOutMax=[]  PParamMin=[]  PParamMax=[]  IParamMin=[]  IParamMax=[]  DParamMin=[]  DParamMax=[]  NParamMin=[]  NParamMax=[]  KbParamMin=[]  KbParamMax=[]  KtParamMin=[]  KtParamMax=[]  KbOutMin=[]  KbOutMax=[]  KtOutMin=[]  KtOutMax=[]  IntegratorOutMin=[]  IntegratorOutMax=[]  FilterOutMin=[]  FilterOutMax=[]  SumI1OutMin=[]  SumI1OutMax=[]  SumI2OutMin=[]  SumI2OutMax=[]  SumI3OutMin=[]  SumI3OutMax=[]  SumI4OutMin=[]  SumI4OutMax=[]  SumDOutMin=[]  SumDOutMax=[]  DifferentiatorOutMin=[]  DifferentiatorOutMax=[]  FilterDiffOutCoefMin=[]  FilterDiffOutCoefMax=[]  ReciprocalOutMin=[]  ReciprocalOutMax=[]  SumDenOutMin=[]  SumDenOutMax=[]  SumNumOutMin=[]  SumNumOutMax=[]  DivideOutMin=[]  DivideOutMax=[]  UdiffTsProdOutMin=[]  UdiffTsProdOutMax=[]  NTsProdOutMin=[]  NTsProdOutMax=[]  UintegralTsProdOutMin=[]  UintegralTsProdOutMax=[]  UngainTsProdOutMin=[]  UngainTsProdOutMax=[]  ClampingZeroOutDataTypeStr=Inherit: Inherit via back propagation  ClampingZeroOutMin=[]  ClampingZeroOutMax=[]  FilterDenConstantOutDataTypeStr=Inherit: Inherit via back propagation  FilterDenConstantOutMin=[]  FilterDenConstantOutMax=[]  PCopyOutDataTypeStr=Inherit: Inherit via back propagation  PCopyOutMin=[]  PCopyOutMax=[]  NCopyOutDataTypeStr=Inherit: Inherit via back propagation  NCopyOutMin=[]  NCopyOutMax=[]  IntegratorContinuousStateAttributes=''  IntegratorStateMustResolveToSignalObject=off  IntegratorRTWStateStorageClass=Auto  FilterContinuousStateAttributes=''  FilterStateMustResolveToSignalObject=off  FilterRTWStateStorageClass=Auto  ParallelPVariant=InternalParameters  IdealPVariant=Disabled  IVariant=Disabled  DVariant=InternalParameters  IntegratorVariant=Disabled  SatVariant=Enabled  AWVariant=Disabled  PCopyVariant=Disabled  TRVariant=Disabled  FdbkBlocksVariant=Forward  IdealPFdbkVariant=Disabled  SatFdbkVariant=Disabled  DerivativeFilterVariant=ContFilter  NVariant=InternalParameters  NCopyVariant=Disabled  FilterICVariant=InternalICsFilter  IntegratorICVariant=Disabled  ExternalResetVariant=Disabled  TRSumVariant=Passthrough  SumFdbkVariant=Disabled  SumVariant=Sum_PD  TsampFilterVariant=InternalTs  TsampNgainVariant=Passthrough  TsampIntegralVariant=Disabled_SignalSpec  ExternalSaturationOutDataTypeStr=Inherit: Same as second input  DerivativeSourceVariant=ErrorSignal  PreIntVariant=InternalPreInt
  PID Controller13 : slpidlib/PID Controller  Commented=on  Controller=PD  Form=Parallel  TimeDomain=Continuous-time  UseExternalTs=off  SampleTime=-1  IntegratorMethod=Forward Euler  FilterMethod=Forward Euler  ControllerParametersSource=internal  P=1  I=1  UseKiTs=off  D=1  UseExternalDerivativeSource=off  N=200  UseFilter=on  TunerSelectOption=Transfer Function Based (PID Tuner App)  InitialConditionSource=internal  InitialConditionForIntegrator=0  InitialConditionForFilter=0  DifferentiatorICPrevScaledInput=0  ExternalReset=none  TrackingMode=off  Kt=1  LimitOutput=on  SatLimitsSource=internal  UpperSaturationLimit=0.5  LowerSaturationLimit=-0.5  LinearizeAsGain=on  AntiWindupMode=none  Kb=1  LimitIntegrator=off  UpperIntegratorSaturationLimit=inf  LowerIntegratorSaturationLimit=-inf  POutMin=[]  POutMax=[]  IOutMin=[]  IOutMax=[]  DOutMin=[]  DOutMax=[]  NOutMin=[]  NOutMax=[]  SumOutMin=[]  SumOutMax=[]  SaturationOutMin=[]  SaturationOutMax=[]  PParamMin=[]  PParamMax=[]  IParamMin=[]  IParamMax=[]  DParamMin=[]  DParamMax=[]  NParamMin=[]  NParamMax=[]  KbParamMin=[]  KbParamMax=[]  KtParamMin=[]  KtParamMax=[]  KbOutMin=[]  KbOutMax=[]  KtOutMin=[]  KtOutMax=[]  IntegratorOutMin=[]  IntegratorOutMax=[]  FilterOutMin=[]  FilterOutMax=[]  SumI1OutMin=[]  SumI1OutMax=[]  SumI2OutMin=[]  SumI2OutMax=[]  SumI3OutMin=[]  SumI3OutMax=[]  SumI4OutMin=[]  SumI4OutMax=[]  SumDOutMin=[]  SumDOutMax=[]  DifferentiatorOutMin=[]  DifferentiatorOutMax=[]  FilterDiffOutCoefMin=[]  FilterDiffOutCoefMax=[]  ReciprocalOutMin=[]  ReciprocalOutMax=[]  SumDenOutMin=[]  SumDenOutMax=[]  SumNumOutMin=[]  SumNumOutMax=[]  DivideOutMin=[]  DivideOutMax=[]  UdiffTsProdOutMin=[]  UdiffTsProdOutMax=[]  NTsProdOutMin=[]  NTsProdOutMax=[]  UintegralTsProdOutMin=[]  UintegralTsProdOutMax=[]  UngainTsProdOutMin=[]  UngainTsProdOutMax=[]  ClampingZeroOutDataTypeStr=Inherit: Inherit via back propagation  ClampingZeroOutMin=[]  ClampingZeroOutMax=[]  FilterDenConstantOutDataTypeStr=Inherit: Inherit via back propagation  FilterDenConstantOutMin=[]  FilterDenConstantOutMax=[]  PCopyOutDataTypeStr=Inherit: Inherit via back propagation  PCopyOutMin=[]  PCopyOutMax=[]  NCopyOutDataTypeStr=Inherit: Inherit via back propagation  NCopyOutMin=[]  NCopyOutMax=[]  IntegratorContinuousStateAttributes=''  IntegratorStateMustResolveToSignalObject=off  IntegratorRTWStateStorageClass=Auto  FilterContinuousStateAttributes=''  FilterStateMustResolveToSignalObject=off  FilterRTWStateStorageClass=Auto  ParallelPVariant=InternalParameters  IdealPVariant=Disabled  IVariant=Disabled  DVariant=InternalParameters  IntegratorVariant=Disabled  SatVariant=Enabled  AWVariant=Disabled  PCopyVariant=Disabled  TRVariant=Disabled  FdbkBlocksVariant=Forward  IdealPFdbkVariant=Disabled  SatFdbkVariant=Disabled  DerivativeFilterVariant=ContFilter  NVariant=InternalParameters  NCopyVariant=Disabled  FilterICVariant=InternalICsFilter  IntegratorICVariant=Disabled  ExternalResetVariant=Disabled  TRSumVariant=Passthrough  SumFdbkVariant=Disabled  SumVariant=Sum_PD  TsampFilterVariant=InternalTs  TsampNgainVariant=Passthrough  TsampIntegralVariant=Disabled_SignalSpec  ExternalSaturationOutDataTypeStr=Inherit: Same as second input  DerivativeSourceVariant=ErrorSignal  PreIntVariant=InternalPreInt
  PID Controller14 : slpidlib/PID Controller  Commented=on  Controller=PD  Form=Parallel  TimeDomain=Continuous-time  UseExternalTs=off  SampleTime=-1  IntegratorMethod=Forward Euler  FilterMethod=Forward Euler  ControllerParametersSource=internal  P=1  I=1  UseKiTs=off  D=1  UseExternalDerivativeSource=off  N=200  UseFilter=on  TunerSelectOption=Transfer Function Based (PID Tuner App)  InitialConditionSource=internal  InitialConditionForIntegrator=0  InitialConditionForFilter=0  DifferentiatorICPrevScaledInput=0  ExternalReset=none  TrackingMode=off  Kt=1  LimitOutput=on  SatLimitsSource=internal  UpperSaturationLimit=0.5  LowerSaturationLimit=-0.5  LinearizeAsGain=on  AntiWindupMode=none  Kb=1  LimitIntegrator=off  UpperIntegratorSaturationLimit=inf  LowerIntegratorSaturationLimit=-inf  POutMin=[]  POutMax=[]  IOutMin=[]  IOutMax=[]  DOutMin=[]  DOutMax=[]  NOutMin=[]  NOutMax=[]  SumOutMin=[]  SumOutMax=[]  SaturationOutMin=[]  SaturationOutMax=[]  PParamMin=[]  PParamMax=[]  IParamMin=[]  IParamMax=[]  DParamMin=[]  DParamMax=[]  NParamMin=[]  NParamMax=[]  KbParamMin=[]  KbParamMax=[]  KtParamMin=[]  KtParamMax=[]  KbOutMin=[]  KbOutMax=[]  KtOutMin=[]  KtOutMax=[]  IntegratorOutMin=[]  IntegratorOutMax=[]  FilterOutMin=[]  FilterOutMax=[]  SumI1OutMin=[]  SumI1OutMax=[]  SumI2OutMin=[]  SumI2OutMax=[]  SumI3OutMin=[]  SumI3OutMax=[]  SumI4OutMin=[]  SumI4OutMax=[]  SumDOutMin=[]  SumDOutMax=[]  DifferentiatorOutMin=[]  DifferentiatorOutMax=[]  FilterDiffOutCoefMin=[]  FilterDiffOutCoefMax=[]  ReciprocalOutMin=[]  ReciprocalOutMax=[]  SumDenOutMin=[]  SumDenOutMax=[]  SumNumOutMin=[]  SumNumOutMax=[]  DivideOutMin=[]  DivideOutMax=[]  UdiffTsProdOutMin=[]  UdiffTsProdOutMax=[]  NTsProdOutMin=[]  NTsProdOutMax=[]  UintegralTsProdOutMin=[]  UintegralTsProdOutMax=[]  UngainTsProdOutMin=[]  UngainTsProdOutMax=[]  ClampingZeroOutDataTypeStr=Inherit: Inherit via back propagation  ClampingZeroOutMin=[]  ClampingZeroOutMax=[]  FilterDenConstantOutDataTypeStr=Inherit: Inherit via back propagation  FilterDenConstantOutMin=[]  FilterDenConstantOutMax=[]  PCopyOutDataTypeStr=Inherit: Inherit via back propagation  PCopyOutMin=[]  PCopyOutMax=[]  NCopyOutDataTypeStr=Inherit: Inherit via back propagation  NCopyOutMin=[]  NCopyOutMax=[]  IntegratorContinuousStateAttributes=''  IntegratorStateMustResolveToSignalObject=off  IntegratorRTWStateStorageClass=Auto  FilterContinuousStateAttributes=''  FilterStateMustResolveToSignalObject=off  FilterRTWStateStorageClass=Auto  ParallelPVariant=InternalParameters  IdealPVariant=Disabled  IVariant=Disabled  DVariant=InternalParameters  IntegratorVariant=Disabled  SatVariant=Enabled  AWVariant=Disabled  PCopyVariant=Disabled  TRVariant=Disabled  FdbkBlocksVariant=Forward  IdealPFdbkVariant=Disabled  SatFdbkVariant=Disabled  DerivativeFilterVariant=ContFilter  NVariant=InternalParameters  NCopyVariant=Disabled  FilterICVariant=InternalICsFilter  IntegratorICVariant=Disabled  ExternalResetVariant=Disabled  TRSumVariant=Passthrough  SumFdbkVariant=Disabled  SumVariant=Sum_PD  TsampFilterVariant=InternalTs  TsampNgainVariant=Passthrough  TsampIntegralVariant=Disabled_SignalSpec  ExternalSaturationOutDataTypeStr=Inherit: Same as second input  DerivativeSourceVariant=ErrorSignal  PreIntVariant=InternalPreInt
  PID Controller9 : slpidlib/PID Controller  Commented=on  Controller=PD  Form=Parallel  TimeDomain=Continuous-time  UseExternalTs=off  SampleTime=-1  IntegratorMethod=Forward Euler  FilterMethod=Forward Euler  ControllerParametersSource=internal  P=1  I=1  UseKiTs=off  D=1  UseExternalDerivativeSource=off  N=200  UseFilter=on  TunerSelectOption=Transfer Function Based (PID Tuner App)  InitialConditionSource=internal  InitialConditionForIntegrator=0  InitialConditionForFilter=0  DifferentiatorICPrevScaledInput=0  ExternalReset=none  TrackingMode=off  Kt=1  LimitOutput=on  SatLimitsSource=internal  UpperSaturationLimit=1  LowerSaturationLimit=-1  LinearizeAsGain=on  AntiWindupMode=none  Kb=1  LimitIntegrator=off  UpperIntegratorSaturationLimit=inf  LowerIntegratorSaturationLimit=-inf  POutMin=[]  POutMax=[]  IOutMin=[]  IOutMax=[]  DOutMin=[]  DOutMax=[]  NOutMin=[]  NOutMax=[]  SumOutMin=[]  SumOutMax=[]  SaturationOutMin=[]  SaturationOutMax=[]  PParamMin=[]  PParamMax=[]  IParamMin=[]  IParamMax=[]  DParamMin=[]  DParamMax=[]  NParamMin=[]  NParamMax=[]  KbParamMin=[]  KbParamMax=[]  KtParamMin=[]  KtParamMax=[]  KbOutMin=[]  KbOutMax=[]  KtOutMin=[]  KtOutMax=[]  IntegratorOutMin=[]  IntegratorOutMax=[]  FilterOutMin=[]  FilterOutMax=[]  SumI1OutMin=[]  SumI1OutMax=[]  SumI2OutMin=[]  SumI2OutMax=[]  SumI3OutMin=[]  SumI3OutMax=[]  SumI4OutMin=[]  SumI4OutMax=[]  SumDOutMin=[]  SumDOutMax=[]  DifferentiatorOutMin=[]  DifferentiatorOutMax=[]  FilterDiffOutCoefMin=[]  FilterDiffOutCoefMax=[]  ReciprocalOutMin=[]  ReciprocalOutMax=[]  SumDenOutMin=[]  SumDenOutMax=[]  SumNumOutMin=[]  SumNumOutMax=[]  DivideOutMin=[]  DivideOutMax=[]  UdiffTsProdOutMin=[]  UdiffTsProdOutMax=[]  NTsProdOutMin=[]  NTsProdOutMax=[]  UintegralTsProdOutMin=[]  UintegralTsProdOutMax=[]  UngainTsProdOutMin=[]  UngainTsProdOutMax=[]  ClampingZeroOutDataTypeStr=Inherit: Inherit via back propagation  ClampingZeroOutMin=[]  ClampingZeroOutMax=[]  FilterDenConstantOutDataTypeStr=Inherit: Inherit via back propagation  FilterDenConstantOutMin=[]  FilterDenConstantOutMax=[]  PCopyOutDataTypeStr=Inherit: Inherit via back propagation  PCopyOutMin=[]  PCopyOutMax=[]  NCopyOutDataTypeStr=Inherit: Inherit via back propagation  NCopyOutMin=[]  NCopyOutMax=[]  IntegratorContinuousStateAttributes=''  IntegratorStateMustResolveToSignalObject=off  IntegratorRTWStateStorageClass=Auto  FilterContinuousStateAttributes=''  FilterStateMustResolveToSignalObject=off  FilterRTWStateStorageClass=Auto  ParallelPVariant=InternalParameters  IdealPVariant=Disabled  IVariant=Disabled  DVariant=InternalParameters  IntegratorVariant=Disabled  SatVariant=Enabled  AWVariant=Disabled  PCopyVariant=Disabled  TRVariant=Disabled  FdbkBlocksVariant=Forward  IdealPFdbkVariant=Disabled  SatFdbkVariant=Disabled  DerivativeFilterVariant=ContFilter  NVariant=InternalParameters  NCopyVariant=Disabled  FilterICVariant=InternalICsFilter  IntegratorICVariant=Disabled  ExternalResetVariant=Disabled  TRSumVariant=Passthrough  SumFdbkVariant=Disabled  SumVariant=Sum_PD  TsampFilterVariant=InternalTs  TsampNgainVariant=Passthrough  TsampIntegralVariant=Disabled_SignalSpec  ExternalSaturationOutDataTypeStr=Inherit: Same as second input  DerivativeSourceVariant=ErrorSignal  PreIntVariant=InternalPreInt
  Sum8 : Sum  Inputs=|+-
  target dpos-dq : Outport
  wires:
  ref pos-q/1 -> Sum8/1
  Demux/3 -> PID Controller11/1
  Demux/6 -> PID Controller14/1
  Demux/5 -> PID Controller13/1
  Demux/2 -> PID Controller10/1
  Demux/4 -> PID Controller12/1
  Demux/1 -> PID Controller9/1
  real pos-q/1 -> Sum8/2
  Sum8/1 -> PID Controller1/1
  PID Controller1/1 -> target dpos-dq/1
